simulink model "controol"  (R2020b)
settings: Solver=VariableStepAuto  StartTime=0.0  StopTime=20  RelTol=1e-3
settings Model: Creator=angello  LastModifiedBy=angello

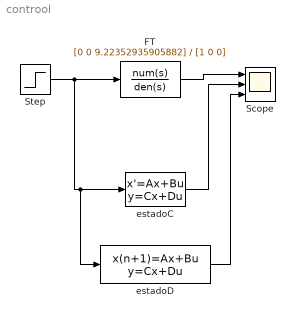
== system controol ==
  FT : TransferFcn  Numerator=[0 0 9.22352935905882]  Denominator=[1 0 0]
  Scope : Scope  NumInputPorts=3
  Step : Step  Time=0  SampleTime=0
  estadoC : StateSpace  A=[0 1;0 0]  B=[0;9.22352935905882]  C=[1 0]  D=0  InitialCondition=0
  estadoD : DiscreteStateSpace  A=[1 19;0 1]  B=[1664.84704931012;175.247057822118]  C=[1 0]  D=0  SampleTime=19
  wires:
  Step/1 -> estadoD/1, estadoC/1, FT/1
  FT/1 -> Scope/1
  estadoC/1 -> Scope/2
  estadoD/1 -> Scope/3
